simulink model "exercise_1"  (R2025a)
settings: Solver=VariableStepAuto  StartTime=0.0  StopTime=10.0  RelTol=1e-3
settings Model: Creator=modeand16864  LastModifiedBy=modeand16864

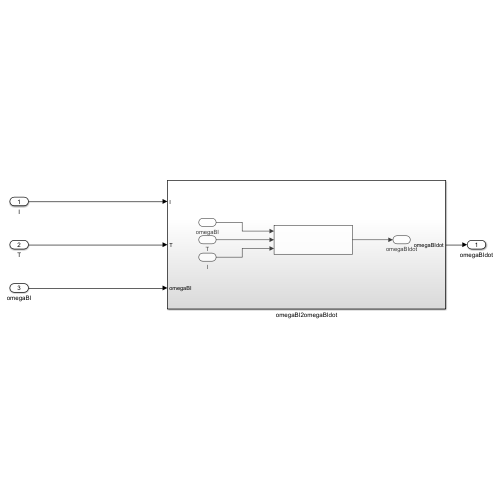
[thumbnail: Simulink's stored preview of the top-level diagram]
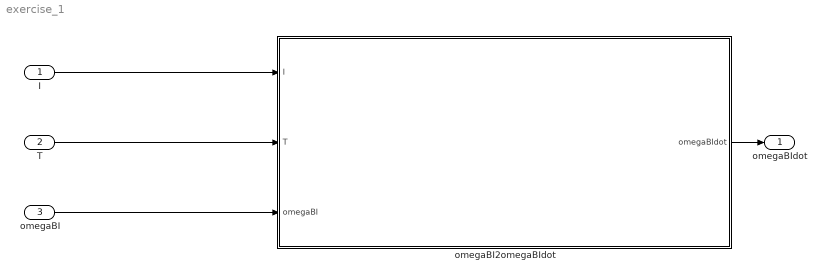
== system exercise_1 ==
  I : Inport
  T : Inport  Port=2
  omegaBI : Inport  Port=3
  omegaBI2omegaBIdot : Subsystem
  omegaBIdot : Outport
  wires:
  I/1 -> omegaBI2omegaBIdot/1(I)
  T/1 -> omegaBI2omegaBIdot/2(T)
  omegaBI/1 -> omegaBI2omegaBIdot/3(omegaBI)
  omegaBI2omegaBIdot/1(omegaBIdot) -> omegaBIdot/1

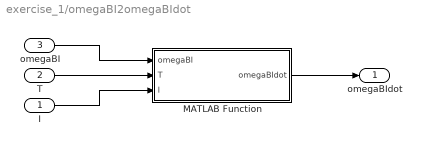
== system exercise_1/omegaBI2omegaBIdot ==
  I : Inport
  T : Inport  Port=2
  omegaBI : Inport  Port=3
  MATLAB Function : MATLAB Function  TreatAsAtomicUnit=on
  omegaBIdot : Outport
  wires:
  I/1 -> MATLAB Function/3(I)
  T/1 -> MATLAB Function/2(T)
  MATLAB Function/1(omegaBIdot) -> omegaBIdot/1
  omegaBI/1 -> MATLAB Function/1(omegaBI)

== matlab function exercise_1/omegaBI2omegaBIdot/MATLAB Function ==
  data: omegaBI input; T input; I input; omegaBIdot output
function omegaBIdot = fcn(omegaBI, T, I)

omegaBIdot = I'*(T-cross(omegaBI, I*omegaBI));
